simulink model "MANUAL_INTEGRATION_TEST_01"  (Simulink 8.1)
settings: Solver=ode4  StartTime=0.0  StopTime=inf  FixedStep=Ts  MaxStep=1e-3  RelTol=1e-3
model workspace (MAT data in the model file):
  op_snapshot1 : opcond.OperatingPoint (value not decoded)
PostLoadFcn:
  | INTEGRATION_TEST_01_init;
InitFcn:
  | INTEGRATION_TEST_01_init;
values from neighbouring files (symbols this model uses):
  CMD_signals = [1 2 3 4 5 6 7 8 9 10 11 12 ... (1568 elements, 49x32)]    [CMD_signals.mat]
undefined symbols (not defined in the file or in its folder): cable_spec, DiscIntNeverNeededParam, fdesignblkfcn, gcbh, Generator, Left, NG_CHP, NG_CHP_lib, NG_Genset_lib, ph, relay_par, SIM_HIL, Ts, type, V
libraries: simulink x29, rtio_opalrt_common x21, rtlab x7, powerlib_extras x7, simulink_extras x7, cables_lib x6, breaker_lib x4, rtio_generic_modbus x4, powerlib x4, rteventslib x4, Load_lib x3, ssn_lib x2
(part 1 of 4)
settings Model: ARTEMISmethode_block_infos=$$__separator__$$MANUAL_INTEGRATION_TEST_01/ARTEMIS Guide$$__separator__$$  Creator=RE25624  LastModifiedBy=RE25624  BufferReuse=off
settings SolverCC: ZeroCrossAlgorithm=Adaptive
settings DataIOCC: ExternalInput=getinputstruct(op_snapshot1)  InitialState=getstatestruct(op_snapshot1)  LimitDataPoints=off  MaxDataPoints=90060  SignalLoggingSaveFormat=Dataset  SaveOutput=off  SignalLogging=off  DSMLogging=off  SaveTime=off  OutputSaveName=result
settings OptimizationCC: BlockReduction=off  OptimizeBlockIOStorage=off  BufferReuse=off  ExpressionFolding=off  LocalBlockOutputs=off
settings DebuggingCC: MaxConsecutiveZCsMsg=warning  IgnoredZcDiagnostic=none  SolverPrmCheckMsg=none  MultiTaskRateTransMsg=warning  FcnCallInpInsideContextMsg=EnableAllAsWarning  FrameProcessingCompatibilityMsg=error  ModelReferenceExtraNoncontSigs=warning  StrictBusMsg=None
settings ModelReferenceCC: UpdateModelReferenceTargets=IfOutOfDate
settings SFSimCC: SFSimEcho=off
settings GRTTargetCC: CodeReplacementLibrary=C89/C90 (ANSI)

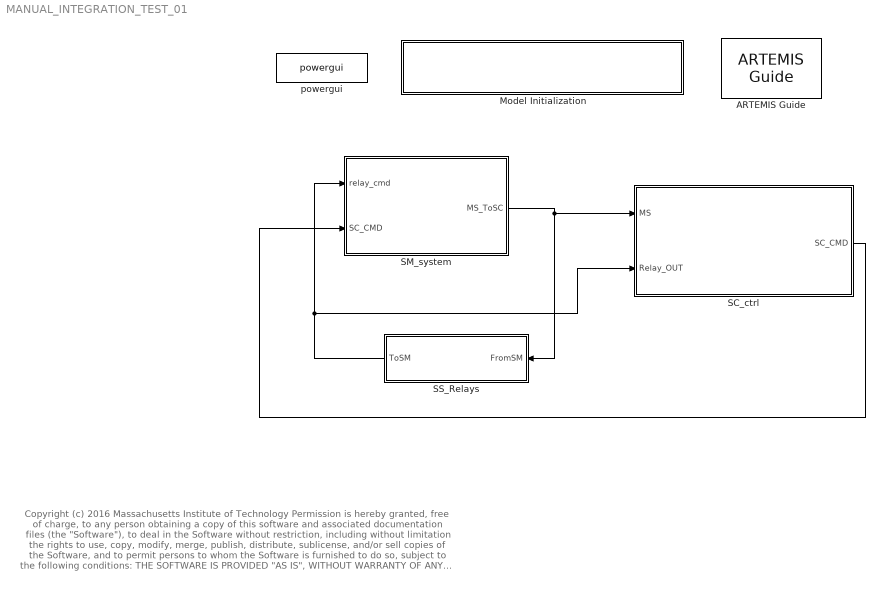
== system MANUAL_INTEGRATION_TEST_01 ==
  note: Copyright (c) 2016 Massachusetts Institute of Technology
      | Permission is hereby granted, free of charge, to any person obtaining a copy of this software and associated documentation files (the "Software"), to deal
      | in the Software without restriction, including without limitation the rights to use, copy, modify, merge, publish, distribute, sublicense, and/or sell copies of the
      | Software, and to permit persons to whom the Software is furnished to do so, subject to the following conditions:
      |
      | THE SOFTWARE IS PROVIDED "AS IS", WITHOUT WARRANTY OF ANY KIND, EXPRESS OR IMPLIED, INCLUDING BUT NOT LIMITED TO THE
      | WARRANTIES OF MERCHANTABILITY, FITNESS FOR A PARTICULAR PURPOSE AND NONINFRINGEMENT. IN NO EVENT SHALL THE AUTHORS
      | OR COPYRIGHT HOLDERS BE LIABLE FOR ANY CLAIM, DAMAGES OR OTHER LIABILITY, WHETHER IN AN ACTION OF CONTRACT, TORT OR
      | OTHERWISE, ARISING FROM, OUT OF OR IN CONNECTION WITH THE SOFTWARE OR THE USE OR OTHER DEALINGS IN THE SOFTWARE.
  ARTEMIS Guide : artemis/ARTEMIS/ARTEMIS Guide  Tag=FTSSmethode_opal_4hx0r99  Description=5.0_z1  lock=on  Ts=Ts  opt=art5  dyna=off  nb_perm=4  RT_fullcomp=off  ssn=on  ssn_itvc=off  ssn_ivic=off  ssn_ext=off  ssn_solver=Art5 with Backward Euler nodal interface  ssn_impulse=off  ssn_quasimpulse=off  ssn_impulse_loop=2  paraExtinctionThy=off  Thy_Impulse=on  dtc=Off  dtc_opt=normal  ao=on  simtype=off  ct_mac=off  lin_mov=off  lsp=[0.001 2]  spike_skip=Disabled  dtc_extra=1  dtc_sws=normal  dtc_pied=0.5  SPSRulesBlock=SPSRules  tre=on  ctmm=off  LF=off  dpl_type=ARTEMiS DPL  rlc_type=off  custom_type=off  para=on  ssn_ImpulseLoopBlockedStateUpdate=2  ssn_mov_iter_number=5  ssn_switch_iter_number=5
  Model Initialization : Subsystem  AncestorBlock=artemis/Tools /Misc/Model Initialization  mask(Model Functions){InitFcnX=INTEGRATION_TEST_01_init;, prel=off, posl=on, inif=on, strf=off}
      mask prompts: InitFcnX "Initialisation"; prel "Preload Function"; posl "PostLoad Function"; inif "InitFcn"; strf "StartFcn"
      mask init:
      | currentBlock = gcb;
      | root = bdroot(currentBlock);
      | 
      | 
      | if ~strcmp(get_param(root,'BlockDiagramType'),'library')
      |     if prel==1
      |         set_param(root, 'PreLoadFcn', InitFcnX);
      |     else
      |         set_param(root, 'PreLoadFcn', '');
      |     end
      |     if inif==1
      |         set_param(root, 'InitFcn', InitFcnX);
      |     else
      |         set_param(root, 'InitFcn', '');
      |     end
      |     if strf==1
      |         set_param(root, 'StartFcn', InitFcnX);
      |     else
      |         set_param(root, 'StartFcn', '');
      |     end
      |     if posl==1
      |         set_param(root, 'PostLoadFcn', InitFcnX);
      |     else
      |         set_param(root, 'PostLoadFcn', '');
      |     end
      | end
      | 
      | pos = get_param(currentBlock, 'Position');
      | width = pos(3) - pos(1); height = pos(4) - pos(2);
      | txt = [ upper(root) '\n' '- InitFcn. . . . . '  get_param(root, 'InitFcn') ];
      settings: CopyFcn=set_param(gcb,'LinkStatus','inactive')
      mask Display: text(5, height*0.5, txt, 'horizontalAlignment', 'left', 'verticalAlignment', 'middle') ;
  SC_ctrl : Subsystem
  SM_system : Subsystem
  SS_Relays : Subsystem
  powergui : powerlib/powergui  Priority=2  SimulationMode=Discrete  SolverType=Tustin  SampleTime=Ts  frequency=60  SPID=off  DisableSnubberDevices=off  DisableRonSwitches=off  DisableVfSwitches=off  SwTol=0  Interpol=off  DisplayEquations=off  frequencyindice=0  Pbase=100e6  ErrMax=1e-4  Iterations=50  UnitsV=kV  UnitsW=MW  FunctionMessages=off  echomessages=off  HookPort=off  EnableUseOfTLC=off  x0status=blocks  RestoreLinks=warning  ResistiveCurrentMeasurement=off  Frange=logspace(0,3,50)  Ylog=off  Xlog=off  ShowGrid=off  save=off  variable=ZData  structure=0  ZoomFFT=on  StartTime=0.0  cycles=2  DisplayStyle=off  fundamental=60  FreqAxis=off  MaxFrequency=1000  frequencyindicesteady=1  RmsSteady=1  display=off  Ts=0  methode=off
  wires:
  SM_system/1(MS_ToSC) -> SC_ctrl/1(MS), SS_Relays/1(FromSM)
  SS_Relays/1(ToSM) -> SM_system/1(relay_cmd), SC_ctrl/2(Relay_OUT)
  SC_ctrl/1(SC_CMD) -> SM_system/2(SC_CMD)

== system MANUAL_INTEGRATION_TEST_01/Model Initialization ==

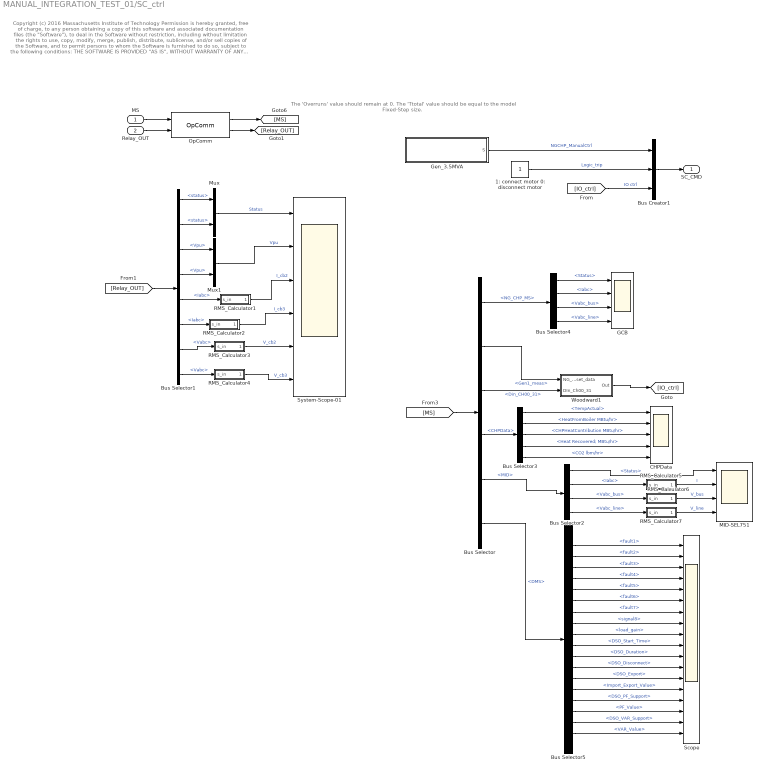
== system MANUAL_INTEGRATION_TEST_01/SC_ctrl ==
  note: The 'Overruns' value should remain at 0.
      | The 'Ttotal' value should be equal to the
      | model Fixed-Step size.
  note: Copyright (c) 2016 Massachusetts Institute of Technology
      | Permission is hereby granted, free of charge, to any person obtaining a copy of this software and associated documentation files (the "Software"), to deal
      | in the Software without restriction, including without limitation the rights to use, copy, modify, merge, publish, distribute, sublicense, and/or sell copies of the
      | Software, and to permit persons to whom the Software is furnished to do so, subject to the following conditions:
      |
      | THE SOFTWARE IS PROVIDED "AS IS", WITHOUT WARRANTY OF ANY KIND, EXPRESS OR IMPLIED, INCLUDING BUT NOT LIMITED TO THE
      | WARRANTIES OF MERCHANTABILITY, FITNESS FOR A PARTICULAR PURPOSE AND NONINFRINGEMENT. IN NO EVENT SHALL THE AUTHORS
      | OR COPYRIGHT HOLDERS BE LIABLE FOR ANY CLAIM, DAMAGES OR OTHER LIABILITY, WHETHER IN AN ACTION OF CONTRACT, TORT OR
      | OTHERWISE, ARISING FROM, OUT OF OR IN CONNECTION WITH THE SOFTWARE OR THE USE OR OTHER DEALINGS IN THE SOFTWARE
  MS : Inport
  Relay_OUT : Inport  Port=2
  1: connect motor 0: disconnect motor : Constant
  Bus Creator1 : BusCreator  Inputs=3
  Bus Selector : BusSelector  OutputSignals=NG_CHP_MS,NG_CHP_MS.Gen1_meas,NG_CHP_MS.Din_CH00_31,NG_CHP_MS.CHPData,MID,DMS
  Bus Selector1 : BusSelector  OutputSignals=CB2.m.status,CB3.m.status,CB2.m.Vpu,CB3.m.Vpu,CB2.m.Iabc,CB3.m.Iabc,CB2.m.Vabc,CB3.m.Vabc
  Bus Selector2 : BusSelector  OutputSignals=Status,Iabc,Vabc_bus,Vabc_line
  Bus Selector3 : BusSelector  OutputSignals=TempActual,HeatFromBoiler MBtu/hr,CHPHeatContribution MBtu/hr,Thermal data.Heat Recovered; MBtu/hr,Thermal data.CO2 lbm/hr
  Bus Selector4 : BusSelector  OutputSignals=NG_CHP_MS.Status,NG_CHP_MS.Iabc,NG_CHP_MS.Vabc_bus,NG_CHP_MS.Vabc_line
  Bus Selector5 : BusSelector  OutputSignals=fault1,fault2,fault3,fault4,fault5,fault6,fault7,signal8,load_gain,DSO_Start_Time,DSO_Duration,DSO_Disconnect,DSO_Export,Import_Export_Value,DSO_PF_Support,PF_Value,DSO_VAR_Support,VAR_Value
  CHPData : Scope  NumInputPorts=5
      settings: ShowLegends=on  TimeRange=10  YMin=20~0~-1~1.37518~932.98  YMax=20.05~5.5~1~1.37533~933.08  SaveName=ScopeData5
  GCB : Scope  NumInputPorts=4
      settings: ShowLegends=on  TimeRange=0.016  YMin=0.95~-800~-12500~-12500  YMax=1.05~800~12500~12500
  Gen_3.5MVA : Subsystem
  MID-SEL751 : Scope  NumInputPorts=4
      settings: ShowLegends=on  TimeRange=0.016  YMin=0.95~-500~-12500~-12500  YMax=1.05~600~12500~12500  SaveName=ScopeData2
  Mux : Mux  Inputs=2
  Mux1 : Mux  Inputs=2
  OpComm : rtlab/OpComm  nbport=2  groupe_acq=1  subsys_rate=0  st=0  Synchronization=on  Interpolation=on  Threshold=1.0  Missed_Data=off  Sim_Time=off  Samples=off  dynSigOut=off  from_console=0  warning_done=off  writeOpCommFile=off  Offset=off
  RMS_Calculator1 : Subsystem
  RMS_Calculator2 : Subsystem
  RMS_Calculator3 : Subsystem
  RMS_Calculator4 : Subsystem
  RMS_Calculator5 : Subsystem
  RMS_Calculator6 : Subsystem
  RMS_Calculator7 : Subsystem
  Scope : Scope  NumInputPorts=18
      settings: YMin=0~0~-1~-1~-1~-1~-1~-1~0.4~0~-5~-5~-5~-5~-5~-5~-5~-5  YMax=1~1~1~1~1~1~1~1~1~4000~5~5~5~5~5~5~5~5  SaveName=ScopeData8  Decimation=100
  System-Scope-01 : Scope  NumInputPorts=6
      settings: ShowLegends=on  TimeRange=1  YMin=0~0~-100~-150~-15000~-15000  YMax=3~1.5~100~150~15000~15000
  Woodward1 : Subsystem
  SC_CMD : Outport
  wires:
  OpComm/1 -> [MS]
  MS/1 -> OpComm/1
  OpComm/2 -> [Relay_OUT]
  Relay_OUT/1 -> OpComm/2
  Woodward1/1(Out) -> [IO_ctrl]
  Bus Selector4/1 -> GCB/1  "<Status>"
  Bus Selector4/2 -> GCB/2  "<Iabc>"
  Bus Selector4/3 -> GCB/3  "<Vabc_bus>"
  Bus Selector4/4 -> GCB/4  "<Vabc_line>"
  Bus Selector/1 -> Bus Selector4/1  "<NG_CHP_MS>"
  Bus Selector/2 -> Woodward1/1(NG_genset_data)  "<Gen1_meas>"
  Bus Selector/3 -> Woodward1/2(DIn_Ch00_31)  "<Din_CH00_31>"
  [MS] -> Bus Selector/1
  Bus Selector/4 -> Bus Selector3/1  "<CHPData>"
  Bus Selector3/1 -> CHPData/1  "<TempActual>"
  Bus Selector3/5 -> CHPData/5  "<CO2 lbm/hr>"
  Bus Selector3/2 -> CHPData/2  "<HeatFromBoiler MBtu/hr>"
  Bus Selector3/3 -> CHPData/3  "<CHPHeatContribution MBtu/hr>"
  Bus Selector3/4 -> CHPData/4  "<Heat Recovered; MBtu/hr>"
  [Relay_OUT] -> Bus Selector1/1
  Bus Selector1/1 -> Mux/1  "<status>"
  Bus Selector1/2 -> Mux/2  "<status>"
  Bus Selector1/3 -> Mux1/1  "<Vpu>"
  Bus Selector1/4 -> Mux1/2  "<Vpu>"
  Bus Creator1/1 -> SC_CMD/1
  1: connect motor 0: disconnect motor/1 -> Bus Creator1/2  "Logic_trip"
  [IO_ctrl] -> Bus Creator1/3  "IO ctrl"
  Gen_3.5MVA/1(S) -> Bus Creator1/1  "NGCHP_ManualCtrl"
  Mux/1 -> System-Scope-01/1  "Status"
  Mux1/1 -> System-Scope-01/2  "Vpu"
  Bus Selector1/5 -> RMS_Calculator1/1(s_in)  "<Iabc>"
  Bus Selector1/6 -> RMS_Calculator2/1(s_in)  "<Iabc>"
  RMS_Calculator1/1(s_out) -> System-Scope-01/3  "I_cb2"
  RMS_Calculator2/1(s_out) -> System-Scope-01/4  "I_cb3"
  Bus Selector1/7 -> RMS_Calculator3/1(s_in)  "<Vabc>"
  Bus Selector1/8 -> RMS_Calculator4/1(s_in)  "<Vabc>"
  RMS_Calculator3/1(s_out) -> System-Scope-01/5  "V_cb2"
  RMS_Calculator4/1(s_out) -> System-Scope-01/6  "V_cb3"
  Bus Selector2/1 -> MID-SEL751/1  "<Status>"
  Bus Selector2/2 -> RMS_Calculator5/1(s_in)  "<Iabc>"
  Bus Selector2/3 -> RMS_Calculator6/1(s_in)  "<Vabc_bus>"
  Bus Selector2/4 -> RMS_Calculator7/1(s_in)  "<Vabc_line>"
  Bus Selector/5 -> Bus Selector2/1  "<MID>"
  RMS_Calculator5/1(s_out) -> MID-SEL751/2  "I"
  RMS_Calculator6/1(s_out) -> MID-SEL751/3  "V_bus"
  RMS_Calculator7/1(s_out) -> MID-SEL751/4  "V_line"
  Bus Selector/6 -> Bus Selector5/1  "<DMS>"
  Bus Selector5/1 -> Scope/1  "<fault1>"
  Bus Selector5/2 -> Scope/2  "<fault2>"
  Bus Selector5/3 -> Scope/3  "<fault3>"
  Bus Selector5/4 -> Scope/4  "<fault4>"
  Bus Selector5/5 -> Scope/5  "<fault5>"
  Bus Selector5/6 -> Scope/6  "<fault6>"
  Bus Selector5/7 -> Scope/7  "<fault7>"
  Bus Selector5/8 -> Scope/8  "<signal8>"
  Bus Selector5/9 -> Scope/9  "<load_gain>"
  Bus Selector5/10 -> Scope/10  "<DSO_Start_Time>"
  Bus Selector5/11 -> Scope/11  "<DSO_Duration>"
  Bus Selector5/12 -> Scope/12  "<DSO_Disconnect>"
  Bus Selector5/13 -> Scope/13  "<DSO_Export>"
  Bus Selector5/14 -> Scope/14  "<Import_Export_Value>"
  Bus Selector5/15 -> Scope/15  "<DSO_PF_Support>"
  Bus Selector5/16 -> Scope/16  "<PF_Value>"
  Bus Selector5/17 -> Scope/17  "<DSO_VAR_Support>"
  Bus Selector5/18 -> Scope/18  "<VAR_Value>"

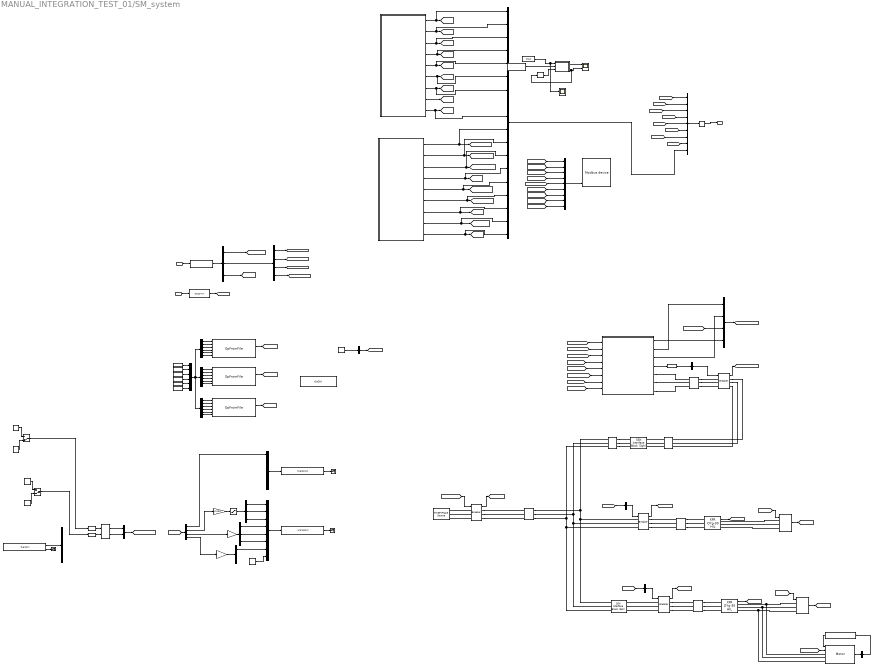
== system MANUAL_INTEGRATION_TEST_01/SM_system ==
  note: Copyright (c) 2016 Massachusetts Institute of Technology
      | Permission is hereby granted, free of charge, to any person obtaining a copy of this software and associated documentation files (the "Software"), to deal
      | in the Software without restriction, including without limitation the rights to use, copy, modify, merge, publish, distribute, sublicense, and/or sell copies of the
      | Software, and to permit persons to whom the Software is furnished to do so, subject to the following conditions:
      |
      | THE SOFTWARE IS PROVIDED "AS IS", WITHOUT WARRANTY OF ANY KIND, EXPRESS OR IMPLIED, INCLUDING BUT NOT LIMITED TO THE
      | WARRANTIES OF MERCHANTABILITY, FITNESS FOR A PARTICULAR PURPOSE AND NONINFRINGEMENT. IN NO EVENT SHALL THE AUTHORS
      | OR COPYRIGHT HOLDERS BE LIABLE FOR ANY CLAIM, DAMAGES OR OTHER LIABILITY, WHETHER IN AN ACTION OF CONTRACT, TORT OR
      | OTHERWISE, ARISING FROM, OUT OF OR IN CONNECTION WITH THE SOFTWARE OR THE USE OR OTHER DEALINGS IN THE SOFTWARE
  note: Stop_index = length of data - 1 to data chopping
  note: This connector also services Genset #2 and  is
      | shared with Genset #1.  Use RJ45 connectors to
      |  intercept Genset #2 I/O (not used in this Device
      | Integration Test) and use for SEL-751
  note: Remove existing connections to Slot 3 I/O, if any
      | ans replace with connections shown below, or use
      | corresponding RJ45 connectors.  (Existing I/O, if any not
      |  used for this Device Integration Test)
  note: This Modbus slave device makes the DMS
      | commands available to the MGC via a Modbus
      | slave
  note: This embedded script updates model
      | parameters and DMS commands based
      | on a predetermined schedule.
  relay_cmd : Inport
  SC_CMD : Inport  Port=2
  200 HP chiller compressor : Load_lib/200 HP chiller compressor
  AnalogOut2 to SEL-751 : rtio_opalrt_common/AnalogOut  CtrlName='OpCtrl'  portNb=4  FcnNos=Slot 2 Module A Subsection 2  size=16  maxcount=8  count=8  numchan=8  israngeinput=off  voltagerange=[ -5 ... 5 ]  slot=1  side=0  mismatch=0  slotside=Slot_2_Module_A
      settings: AttributesFormatString=%<CtrlName>
  Bus Creator : BusCreator  Inputs=9
  Bus Creator1 : BusCreator
  Bus Creator2 : BusCreator  Inputs=1
  Bus Creator3 : BusCreator  Inputs=1
  Bus Creator4 : BusCreator  Inputs=2
  Bus Creator5 : BusCreator  Inputs=18
  Bus Selector1 : BusSelector  OutputSignals=CB2
  Bus Selector2 : BusSelector  OutputSignals=CB3
  Bus Selector3 : BusSelector  OutputSignals=NGCHP_ManualCtrl,IO ctrl,Logic_trip
  Bus Selector4 : BusSelector  OutputSignals=Status,Iabc,Vabc_line,Vabc_bus
  Bus Selector5 : BusSelector  OutputSignals=Woodward,manual_controls,DOUT GR3,DOUT GR3.16 DOUT GR3.CHP_SIM_Cmds
  Bus Selector6 : BusSelector  OutputSignals=RPM
  CB closed : Constant
  CB1-GCB1 : breaker_lib/Breaker  Ts=Ts  mech_delay=cb_mech_delay
  CB2 : breaker_lib/Breaker  Ts=Ts  mech_delay=cb_mech_delay
  CB3 : breaker_lib/Breaker  Ts=Ts  mech_delay=cb_mech_delay
  CT Ratio : Gain  Gain=5/1250
  Cal : Constant  Value=0
  Constant : Constant
  Constant1 : Constant  Value=0
  Constant2 : Constant
  Constant3 : Constant  Value=0
  DMS Modbus  device : rtio_generic_modbus/Modbus device  conf_name=DMS_slave_cfg.opal  conf_name_mask=DMS_slave_cfg.xls  sample_time=0
  DMSCommandsToMGC : Subsystem  mask{DSO_Start_Time=3600, DSO_Duration=0, DSO_Disconnect=1, DSO_Export=0, Import_Export_Value=0, DSO_PF_Support=0, PF_Value=0, DSO_VAR_Support=0, VAR_Value=0}
      mask prompts: DSO_Start_Time "DSO Start Time"; DSO_Duration "DSO Duration"; DSO_Disconnect "DSO Disconnect"; DSO_Export "DSO Export (1) or Import (0)"; Import_Export_Value "Import/Export Value, kW"; DSO_PF_Support "DSO PF Support (1) or Not (0)"; PF_Value "PF Value, pu, "+"(lagging) "-" (leading)"; DSO_VAR_Support "DSO VAR Support (1) or Not (0)"; VAR_Value "Import/Export Value, kVAr"
  Data Type Conversion : DataTypeConversion
  Data Type Conversion1 : DataTypeConversion
  Demux : Demux  Outputs=3
  Demux1 : Demux  Outputs=6
  Demux2 : Demux  Outputs=6
  Demux3 : Demux  Outputs=6
  Demux4 : Demux  Outputs=3
  Demux5 : Demux  Outputs=3
  Demux6 : Demux  Outputs=8
  Digital Clock : DigitalClock  SampleTime=Ts
  DigitalIn from SEL-751 : rtio_opalrt_common/DigitalIn  CtrlName='OpCtrl'  portNb=6  FcnNos=Slot 3 Module A Subsection 2  size=1  maxcount=8  count=8  sampleTime=Ts  numchan=8
      settings: AttributesFormatString=%<CtrlName>
  DigitalOut to SEL-751 : rtio_opalrt_common/DigitalOut  CtrlName='OpCtrl'  portNb=6  FcnNos=Slot 3 Module B Subsection 2  size=1  maxcount=8  count=8  numchan=8
      settings: AttributesFormatString=%<CtrlName>
  Dynamic_Load_1 : Load_lib/Dynamic_Load  V=4160  Ts=Ts
  Dynamic_Load_2 : Load_lib/Dynamic_Load  V=480  Ts=Ts
  Fcn : Fcn  Expr=u(1)==1
  GRID : powerlib/Electrical Sources/Three-Phase Source  Voltage=13800  PhaseAngle=0  Frequency=60  InternalConnection=Yg  SpecifyImpedance=on  Resistance=0.8929  Inductance=16.58e-3  ShortCircuitLevel=375e6  BaseVoltage=13800  XRratio=4.6  BusType=swing  Pref=0  Qref=0  Qmin=-inf  Qmax=inf
  "Interpolation " : Constant
  MID : breaker_lib/Breaker  Ts=Ts  mech_delay=cb_mech_delay
  Manual Switch : ManualSwitch  CurrentSetting=0
  Manual Switch1 : ManualSwitch  CurrentSetting=0
  Memory : Memory
  Memory1 : Memory  X0=1
  Motor : Motor_InductionMachine_lib/Motor
  Mux : Mux  Inputs=6
  Mux1 : Mux  Inputs=8
  Mux2 : Mux  Inputs=9
  Mux4 : Mux  Inputs=8
  NG_CHP1 : Subsystem  AncestorBlock=NG_CHP_lib/NG_CHP
  OpComm : rtlab/OpComm  nbport=1  groupe_acq=1  subsys_rate=0  st=0  Synchronization=on  Interpolation=on  Threshold=1.0  Missed_Data=off  Sim_Time=off  Samples=off  dynSigOut=off  from_console=0  warning_done=off  writeOpCommFile=off  Offset=off
  OpComm2 : rtlab/OpComm  nbport=1  groupe_acq=1  subsys_rate=0  st=0  Synchronization=on  Interpolation=on  Threshold=1.0  Missed_Data=off  Sim_Time=off  Samples=off  dynSigOut=off  from_console=1  warning_done=off  writeOpCommFile=off  Offset=off
  OpCtrl : rtio_opalrt_common/OpCtrl  CtrlName='OpCtrl'  boardid=0  BitstreamFilename=VC707_2-EX-0001-2_2_6_61-32AIO16DIO16DIOSel-01-01.bin  numconfig=-1  mode=Master  externalClock=off  decimRtsi=0  calibIO=off  SampleTime=0  loadinport=-1  BoardType=VC707  SecondaryPresent=off  sync_type=Audio
  OpFromFile : rtlab/DataLogging/OpFromFile  filename_mode=Static (same filename all the time)  reload_mode=Next time model is paused (Real-Time)  init_file_id=0  filename=HeatLoad.mat  rtpath='./'  nrtpath='.\'  sample_time=Ts
  OpFromFile1 : rtlab/DataLogging/OpFromFile  filename_mode=Static (same filename all the time)  reload_mode=Next time model is paused (Real-Time)  init_file_id=0  filename=one_min_data.mat  rtpath='./'  nrtpath='.\'  sample_time=0
  OpFromFile2 : rtlab/DataLogging/OpFromFile  filename_mode=Static (same filename all the time)  reload_mode=Next time model is paused (Real-Time)  init_file_id=0  filename=one_min_data.mat  rtpath='./'  nrtpath='.\'  sample_time=0
  PI-Section : cables_lib/PI-Section  cable_spec=[cable_spec(13, :)]  line_length=5500  parallel_sets=1
  PI-Section1 : cables_lib/PI-Section  cable_spec=[cable_spec(11, :)]  line_length=10  parallel_sets=1
  PI-Section2 : cables_lib/PI-Section  cable_spec=[cable_spec(11, :)]  line_length=2000  parallel_sets=1
  PI-Section3 : cables_lib/PI-Section  cable_spec=[cable_spec(13, :)]  line_length=1500  parallel_sets=1
  PI-Section4 : cables_lib/PI-Section  cable_spec=[cable_spec(13, :)]  line_length=2000  parallel_sets=1
  PI-Section5 : cables_lib/PI-Section  cable_spec=[cable_spec(11, :)]  line_length=10  parallel_sets=1
  PT Ratio1 : Gain  Gain=1/1800
  PT Ratio2 : Gain  Gain=1/1800
  "Repetative " : Constant
  S-R Flip-Flop : simulink_extras/Flip Flops/S-R Flip-Flop  initial_condition=1
  SSN Interface Block (3ph) : ssn_lib/SSN Interface Block (3ph)  nb_phase=3  nb_port=2  p1_type=V-type(Left)  p2_type=V-type (Right)  p3_type=V-type(Left)  p4_type=V-type(Left)  p5_type=V-type(Left)  p6_type=V-type(Left)  p7_type=V-type(Left)  p8_type=V-type(Left)  p9_type=V-type(Left)  p10_type=V-type(Left)  p11_type=V-type(Left)  p12_type=V-type(Left)  p13_type=V-type(Left)  p14_type=V-type(Left)  p15_type=V-type(Left)  p16_type=V-type(Left)  I_port_shunt_resistance=1e9
  SSN Interface Block (3ph)1 : ssn_lib/SSN Interface Block (3ph)  nb_phase=3  nb_port=2  p1_type=V-type(Left)  p2_type=V-type (Right)  p3_type=V-type(Left)  p4_type=V-type(Left)  p5_type=V-type(Left)  p6_type=V-type(Left)  p7_type=V-type(Left)  p8_type=V-type(Left)  p9_type=V-type(Left)  p10_type=V-type(Left)  p11_type=V-type(Left)  p12_type=V-type(Left)  p13_type=V-type(Left)  p14_type=V-type(Left)  p15_type=V-type(Left)  p16_type=V-type(Left)  I_port_shunt_resistance=1e9
  Scheduler : MATLAB Function  TreatAsAtomicUnit=on
  Scope1 : Scope
      settings: YMin=1.04083e-17  YMax=0.2  SaveName=ScopeData6
  Scope4 : Scope  NumInputPorts=3
      settings: YMin=-5~-5~-5  YMax=5~5~5  SaveName=ScopeData7
  "Start_Index " : Constant
  "State " : Constant
  "Stop_Index " : Constant  Value=1800-1
  Terminator : Terminator
  Terminator1 : Terminator
  Terminator2 : Terminator
  Test Sequence Inputs : Constant  Value=CMD_signals
  TestSequenceCommands : Subsystem  mask{fault1=0, fault2=0, fault3=0, fault4=0, fault5=0, fault6=0, fault7=0, fault8=0, load_gain=0.5}
      mask prompts: load_gain "Loads"
  Thermal Protection for Transconductance Amp : Saturate  UpperLimit=5  LowerLimit=-5
  "Time_Scale_Factor " : Constant
  XFR DYg-30 HIL1 : transformer_lib/XFR DYg-30 HIL  Rating=3750  Vp=13800  Vs=4160  Z=4.75  XR=11.4
  XFR DYg-30 HIL2 : transformer_lib/XFR DYg-30 HIL  Rating=2500  Vp=13800  Vs=480  Z=5.75  XR=6.6
  MS_ToSC : Outport
  wires:
  MID/1 -> [MID]
  Bus Creator/1 -> Memory/1
  OpComm/1 -> [relay_cmd]
  relay_cmd/1 -> OpComm/1
  CB1-GCB1/1 -> [NG_CHP_GCB]
  SC_CMD/1 -> OpComm2/1
  Bus Selector5/1 -> [woodward]  "<Woodward>"
  Bus Selector5/3 -> [Dout_GR3]  "<DOUT GR3>"
  Bus Selector5/2 -> [brkcont]  "<manual_controls>"
  [NG_CHP_GCB] -> Bus Creator1/3  "NG_CHP_MS"
  NG_CHP1/3(Generator Data) -> Bus Creator1/2  "Gen1_meas"
  NG_CHP1/2(Out2) -> Bus Creator1/1  "Din_CH00_31"
  XFR DYg-30 HIL1/1 -> [XFR_01]
  "Stop_Index "/1 -> Mux/4
  Demux1/2 -> OpFromFile1/2
  Demux1/5 -> OpFromFile1/5
  OpFromFile1/2 -> [PQLOAD_2]
  "Interpolation "/1 -> Mux/6
  Demux1/4 -> OpFromFile1/4
  Demux1/1 -> OpFromFile1/1
  Demux1/6 -> OpFromFile1/6
  Demux1/3 -> OpFromFile1/3
  "Start_Index "/1 -> Mux/3
  "Time_Scale_Factor "/1 -> Mux/5
  "Repetative "/1 -> Mux/2
  "State "/1 -> Mux/1
  [Dout_GR3] -> NG_CHP1/2(Digital Outputs)
  [brkcont] -> NG_CHP1/3(Console Breakers)
  [woodward] -> NG_CHP1/4(Woodward Enable)
  [NGCHP_MNCTLR] -> NG_CHP1/5(Manual Control (opt))
  [NG_CHP_GCB] -> NG_CHP1/6(GCB)
  [MID] -> NG_CHP1/7(MCB)
  NG_CHP1/1(Out1) -> Bus Creator1/4  "CHPData"
  NG_CHP1/4(GCB Control) -> Fcn/1
  Bus Selector5/4 -> [CHP_SIM_cmds]  "<CHP_SIM_Cmds>"
  OpFromFile/2 -> [heat_load]  "Heat Load MBtu/hr"
  [heat_load] -> NG_CHP1/1(In1)
  [CHP_SIM_cmds] -> NG_CHP1/8(In2)
  Demux2/2 -> OpFromFile/2
  Demux2/5 -> OpFromFile/5
  Demux2/4 -> OpFromFile/4
  Demux2/1 -> OpFromFile/1
  Demux2/6 -> OpFromFile/6
  Demux2/3 -> OpFromFile/3
  Dynamic_Load_1/1 -> [LOAD_1]
  XFR DYg-30 HIL2/1 -> [XFR_02]
  Dynamic_Load_2/1 -> [LOAD_2]
  Bus Creator2/1 -> [cb_c]
  CB closed/1 -> Bus Creator2/1  "Logic_trip"
  CB2/1 -> [CB2]
  CB3/1 -> [CB3]
  [XFR_02] -> Bus Creator/7  "XFR_02"
  [LOAD_2] -> Bus Creator/5  "LOAD_2"
  [XFR_01] -> Bus Creator/6  "XFR_01"
  [MID] -> Bus Creator/1  "MID"
  [CB3] -> Bus Creator/3  "CB3"
  [CB2] -> Bus Creator/2  "CB2"
  [LOAD_1] -> Bus Creator/4  "LOAD_1"
  Bus Creator1/1 -> [NG_CHP_MS]
  [NG_CHP_MS] -> Bus Creator/8  "NG_CHP_MS"
  Demux3/2 -> OpFromFile2/2
  Demux3/5 -> OpFromFile2/5
  OpFromFile2/2 -> [PQLOAD_1]
  Demux3/4 -> OpFromFile2/4
  Demux3/1 -> OpFromFile2/1
  Demux3/6 -> OpFromFile2/6
  Demux3/3 -> OpFromFile2/3
  Mux/1 -> Demux3/1, Demux2/1, Demux1/1
  [PQLOAD_1] -> Dynamic_Load_1/1
  [PQLOAD_2] -> Dynamic_Load_2/1
  [relay_cmd] -> Bus Selector1/1
  Bus Selector1/1 -> CB2/1  "<CB2>"
  [relay_cmd] -> Bus Selector2/1
  Bus Selector2/1 -> CB3/1  "<CB3>"
  Fcn/1 -> Bus Creator3/1  "Logic_trip"
  Bus Creator3/1 -> CB1-GCB1/1  "Logic_trip"
  [SEL751_1_from] -> MID/1
  [motor_cmd] -> Motor/2
  Motor/1 -> Bus Selector6/1
  Bus Selector6/1 -> 200 HP chiller compressor/1  "<RPM>"
  200 HP chiller compressor/1 -> Motor/1
  OpComm2/1 -> Bus Selector3/1
  Bus Selector3/1 -> [NGCHP_MNCTLR]  "<NGCHP_ManualCtrl>"
  Bus Selector3/2 -> Bus Selector5/1  "<IO ctrl>"
  Bus Selector3/3 -> [motor_cmd]  "<Logic_trip>"
  Bus Selector4/2 -> CT Ratio/1  "<Iabc>"
  Demux4/1 -> Mux1/4  "Va"
  Demux4/2 -> Mux1/5  "Vb"
  Demux4/3 -> Mux1/6  "Vc"
  Bus Selector4/4 -> PT Ratio2/1  "<Vabc_bus>"
  Demux5/1 -> Mux1/7  "Vs"
  Bus Selector4/3 -> PT Ratio1/1  "<Vabc_line>"
  Cal/1 -> Mux1/8
  AnalogOut2 to SEL-751/1 -> Terminator/1
  DigitalIn from SEL-751/1 -> Demux6/1
  Manual Switch/1 -> Data Type Conversion/1  "OUT103 Brkr trip"
  Manual Switch1/1 -> Data Type Conversion1/1  "OUT102 Brkr reset"
  Data Type Conversion/1 -> S-R Flip-Flop/1
  Data Type Conversion1/1 -> S-R Flip-Flop/2
  S-R Flip-Flop/1 -> Bus Creator4/1  "Logic_trip"
  S-R Flip-Flop/2 -> Bus Creator4/2  "Logic_reset"
  Bus Selector4/1 -> Mux4/1  "<Status>"
  Mux4/1 -> DigitalOut to SEL-751/1
  DigitalOut to SEL-751/1 -> Terminator1/1
  DigitalIn from SEL-751/2 -> Terminator2/1
  Mux1/1 -> AnalogOut2 to SEL-751/1
  Demux/1 -> Mux1/1  "Ia"
  Demux/3 -> Mux1/3  "Ic"
  Demux/2 -> Mux1/2  "Ib"
  Bus Creator4/1 -> [SEL751_1_from]
  [MID] -> Bus Selector4/1
  Memory/1 -> MS_ToSC/1
  Constant1/1 -> Manual Switch/2
  Constant/1 -> Manual Switch/1
  Constant3/1 -> Manual Switch1/2
  Constant2/1 -> Manual Switch1/1
  Mux2/1 -> DMS Modbus  device/4
  Scheduler/1(y) -> Scope4/1
  Scheduler/2(n1) -> Memory1/1, Scope4/3
  Memory1/1 -> Scheduler/3(n)
  Test Sequence Inputs/1 -> Scheduler/2(CMD_signals)
  Digital Clock/1 -> Scheduler/1(u), Scope1/1
  DMSCommandsToMGC/3(DSO_Disconnect) -> Bus Creator5/12, [DSO_Disconnect]
  DMSCommandsToMGC/4(DSO_Export) -> Bus Creator5/13, [DSO_Export]
  DMSCommandsToMGC/7(PF_Value) -> [PF_Value], Bus Creator5/16
  DMSCommandsToMGC/1(DSO_Start_Time) -> [DSO_Start_Time], Bus Creator5/10
  DMSCommandsToMGC/5(Import_Export_Value) -> Bus Creator5/14, [Import_Export_Value]
  [DSO_Start_Time] -> Mux2/1
  [DSO_Duration] -> Mux2/2
  [DSO_Disconnect] -> Mux2/3
  [DSO_Export] -> Mux2/4
  [Import_Export_Value] -> Mux2/5
  [DSO_PF_Support] -> Mux2/6
  [PF_Value] -> Mux2/7
  [DSO_VAR_Support] -> Mux2/8
  [VAR_Value] -> Mux2/9
  TestSequenceCommands/1(Fault1) -> Bus Creator5/1, [fault1]  "fault1"
  TestSequenceCommands/2(Fault2) -> Bus Creator5/2, [fault2]  "fault2"
  TestSequenceCommands/3(Fault3) -> Bus Creator5/3, [fault3]  "fault3"
  TestSequenceCommands/4(Fault4) -> Bus Creator5/4, [fault4]  "fault4"
  TestSequenceCommands/6(Fault6) -> Bus Creator5/6, [fault6]  "fault6"
  TestSequenceCommands/7(Fault7) -> Bus Creator5/7, [fault7]  "fault7"
  TestSequenceCommands/9(loads) -> Bus Creator5/9, [load_gain]  "load_gain"
  TestSequenceCommands/5(Fault5) -> Bus Creator5/5, [fault5]  "fault5"
  DMSCommandsToMGC/2(DSO_Duration) -> Bus Creator5/11, [DSO_Duration]
  DMSCommandsToMGC/6(DSO_PF_Support) -> Bus Creator5/15, [DSO_PF_Support]
  DMSCommandsToMGC/8(DSO_VAR_Support) -> Bus Creator5/17, [DSO_VAR_Support]
  DMSCommandsToMGC/9(VAR_Value) -> Bus Creator5/18, [VAR_Value]
  Bus Creator5/1 -> Bus Creator/9  "DMS"
  TestSequenceCommands/8("Fault8 ") -> [fault8]  "fault8"
  CT Ratio/1 -> Thermal Protection for Transconductance Amp/1
  PT Ratio1/1 -> Demux4/1
  PT Ratio2/1 -> Demux5/1
  Thermal Protection for Transconductance Amp/1 -> Demux/1
  connections:
  Dynamic_Load_1/LConn1 -- XFR DYg-30 HIL1/RConn1
  Dynamic_Load_1/LConn2 -- XFR DYg-30 HIL1/RConn2
  Dynamic_Load_1/LConn3 -- XFR DYg-30 HIL1/RConn3
  CB2/RConn2 -- PI-Section3/LConn2
  CB2/RConn1 -- PI-Section3/LConn1
  CB2/RConn3 -- PI-Section3/LConn3
  CB3/RConn2 -- PI-Section4/LConn2
  CB3/RConn1 -- PI-Section4/LConn1
  CB3/RConn3 -- PI-Section4/LConn3
  CB3/LConn2 -- SSN Interface Block (3ph)/RConn2
  CB3/LConn1 -- SSN Interface Block (3ph)/RConn1
  CB3/LConn3 -- SSN Interface Block (3ph)/RConn3
  PI-Section5/LConn3 -- PI-Section/RConn3 -- SSN Interface Block (3ph)/LConn3 -- CB2/LConn3
  PI-Section5/LConn2 -- PI-Section/RConn2 -- SSN Interface Block (3ph)/LConn2 -- CB2/LConn2
  PI-Section5/LConn1 -- PI-Section/RConn1 -- SSN Interface Block (3ph)/LConn1 -- CB2/LConn1
  Dynamic_Load_2/LConn1 -- Motor/LConn1 -- XFR DYg-30 HIL2/RConn1
  Dynamic_Load_2/LConn3 -- Motor/LConn3 -- XFR DYg-30 HIL2/RConn3
  Dynamic_Load_2/LConn2 -- Motor/LConn2 -- XFR DYg-30 HIL2/RConn2
  PI-Section4/RConn1 -- XFR DYg-30 HIL2/LConn1
  PI-Section4/RConn2 -- XFR DYg-30 HIL2/LConn2
  PI-Section4/RConn3 -- XFR DYg-30 HIL2/LConn3
  PI-Section3/RConn2 -- XFR DYg-30 HIL1/LConn2
  PI-Section3/RConn3 -- XFR DYg-30 HIL1/LConn3
  PI-Section3/RConn1 -- XFR DYg-30 HIL1/LConn1
  PI-Section2/RConn3 -- CB1-GCB1/LConn3
  PI-Section2/RConn2 -- CB1-GCB1/LConn2
  PI-Section2/RConn1 -- CB1-GCB1/LConn1
  NG_CHP1/RConn2 -- PI-Section2/LConn2
  NG_CHP1/RConn3 -- PI-Section2/LConn3
  NG_CHP1/RConn1 -- PI-Section2/LConn1
  PI-Section1/LConn1 -- SSN Interface Block (3ph)1/RConn1
  PI-Section1/LConn2 -- SSN Interface Block (3ph)1/RConn2
  PI-Section1/LConn3 -- SSN Interface Block (3ph)1/RConn3
  PI-Section5/RConn2 -- SSN Interface Block (3ph)1/LConn2
  PI-Section5/RConn1 -- SSN Interface Block (3ph)1/LConn1
  PI-Section5/RConn3 -- SSN Interface Block (3ph)1/LConn3
  CB1-GCB1/RConn3 -- PI-Section1/RConn3
  CB1-GCB1/RConn1 -- PI-Section1/RConn1
  CB1-GCB1/RConn2 -- PI-Section1/RConn2
  MID/RConn3 -- PI-Section/LConn3
  MID/RConn2 -- PI-Section/LConn2
  MID/RConn1 -- PI-Section/LConn1
  MID/LConn3 -- GRID/RConn3
  MID/LConn1 -- GRID/RConn1
  MID/LConn2 -- GRID/RConn2

== system MANUAL_INTEGRATION_TEST_01/SS_Relays ==
  note: Copyright (c) 2016 Massachusetts Institute of Technology
      | Permission is hereby granted, free of charge, to any person obtaining a copy of this software and associated documentation files (the "Software"), to deal
      | in the Software without restriction, including without limitation the rights to use, copy, modify, merge, publish, distribute, sublicense, and/or sell copies of the
      | Software, and to permit persons to whom the Software is furnished to do so, subject to the following conditions:
      |
      | THE SOFTWARE IS PROVIDED "AS IS", WITHOUT WARRANTY OF ANY KIND, EXPRESS OR IMPLIED, INCLUDING BUT NOT LIMITED TO THE
      | WARRANTIES OF MERCHANTABILITY, FITNESS FOR A PARTICULAR PURPOSE AND NONINFRINGEMENT. IN NO EVENT SHALL THE AUTHORS
      | OR COPYRIGHT HOLDERS BE LIABLE FOR ANY CLAIM, DAMAGES OR OTHER LIABILITY, WHETHER IN AN ACTION OF CONTRACT, TORT OR
      | OTHERWISE, ARISING FROM, OUT OF OR IN CONNECTION WITH THE SOFTWARE OR THE USE OR OTHER DEALINGS IN THE SOFTWARE
  FromSM : Inport
  Bus Creator : BusCreator  Inputs=2
  Bus Selector : BusSelector  OutputSignals=CB2,CB3
  Generic_Relay_v2_1 : relay_modbus_lib/Generic_Relay_v2_1  Ts=Ts  relay_settings=[relay_par(1,:)]
  Generic_Relay_v2_2 : relay_modbus_lib/Generic_Relay_v2_1  Ts=Ts  relay_settings=[relay_par(2,:)]
  Memory : Memory
  Modbus device : rtio_generic_modbus/Modbus device  conf_name=F1_relay_cfg1.opal  conf_name_mask=F1_relay_cfg1.xls  sample_time=Ts
  Modbus device1 : rtio_generic_modbus/Modbus device  conf_name=F1_relay_cfg2.opal  conf_name_mask=F1_relay_cfg2.xls  sample_time=Ts
  OpComm : rtlab/OpComm  nbport=1  groupe_acq=1  subsys_rate=0  st=0  Synchronization=on  Interpolation=on  Threshold=1.0  Missed_Data=off  Sim_Time=off  Samples=off  dynSigOut=off  from_console=0  warning_done=off  writeOpCommFile=off  Offset=off
  ToSM : Outport
  wires:
  OpComm/1 -> Bus Selector/1
  FromSM/1 -> OpComm/1
  Generic_Relay_v2_1/1 -> Bus Creator/1  "CB2"
  Generic_Relay_v2_2/1 -> Bus Creator/2  "CB3"
  Bus Creator/1 -> Memory/1
  Modbus device/1 -> Generic_Relay_v2_1/2
  Generic_Relay_v2_1/2 -> Modbus device/1
  Modbus device1/1 -> Generic_Relay_v2_2/2
  Generic_Relay_v2_2/2 -> Modbus device1/1
  Bus Selector/2 -> Generic_Relay_v2_2/1  "<CB3>"
  Bus Selector/1 -> Generic_Relay_v2_1/1  "<CB2>"
  Memory/1 -> ToSM/1

== system MANUAL_INTEGRATION_TEST_01/SC_ctrl/Gen_3.5MVA ==
  1 - PQ 2 - PV 3 - VF : Constant  Value=3
  2.5 - 130 s : DiscretePulseGenerator  Period=150/Ts  PulseWidth=127.5/Ts  PhaseDelay=2.5/Ts  SampleTime=Ts
  Bus Creator : BusCreator  Inputs=6
  DONOTCHANGE : Constant
  Enable = 1 Disable = 0 : Constant  Value=0
  F : simulink/Math Operations/Slider Gain  low=0.97  gain=1  high=1.03
  Fcmd pu 1.005 - 1.03 : Constant  Value=1.005
  P : simulink/Math Operations/Slider Gain  low=0  gain=0.8  high=1.1
  Pfactor : Gain  Gain=.9
  Q : simulink/Math Operations/Slider Gain  low=0.01  gain=0.2  high=0.4
  Qfactor : Gain  Gain=.43
  S Profile : simulink/Sources/Repeating Sequence Stair  OutValues=[.1 .1 .1 .1 .1 .1 .5 .5 .5 .5 .5 .5 .5 .5 .5 .5 .5 .5 1 1 1 1 1 ]  tsamp=[5 Ts]  OutMin=[]  OutMax=[]  OutDataTypeStr=Inherit: Inherit via back propagation  OutDataType=fixdt(0,8)  ConRadixGroup=Best Precision: Vector-wise  OutScaling=2^-12
  V : simulink/Math Operations/Slider Gain  low=0.9  gain=1  high=1.1
  VF - to end : simulink/Sources/Repeating Sequence Stair  OutValues=[3 3 3 3 3 3 3 3 3 3 3 3 3 3 3 3 3 3 3 3 3 3 3 3 3 3 3 3 3 3 3 ]  tsamp=[5 Ts]  OutMin=[]  OutMax=[]  OutDataTypeStr=Inherit: Inherit via back propagation  OutDataType=fixdt(0,8)  ConRadixGroup=Best Precision: Vector-wise  OutScaling=2^-12
  Vcmd pu 1.005 - 1.01 : Constant  Value=1.005
  S : Outport
  wires:
  Pfactor/1 -> Bus Creator/1  "P"
  Fcmd pu 1.005 - 1.03/1 -> Bus Creator/4  "F"
  2.5 - 130 s/1 -> Bus Creator/6  "Enable"
  VF - to end/1 -> Bus Creator/5  "Mode"
  Vcmd pu 1.005 - 1.01/1 -> Bus Creator/3  "V"
  Qfactor/1 -> Bus Creator/2  "Q"
  S Profile/1 -> Pfactor/1, Qfactor/1  "P"
  Bus Creator/1 -> S/1
  DONOTCHANGE/1 -> F/1, V/1, Q/1, P/1

== system MANUAL_INTEGRATION_TEST_01/SC_ctrl/RMS_Calculator1 ==
  s_in : Inport
  Demux : Demux  Outputs=3
  Discrete  Mean value6 : powerlib_extras/Discrete Measurements/Discrete  Mean value  Freq=60  Vinit=0  Ts=Ts
  Mux2 : Mux  Inputs=2
  Product3 : Product  RndMeth=Zero
  Signed Sqrt : Sqrt  SaturateOnIntegerOverflow=on
  s_out : Outport
  wires:
  Demux/1 -> Product3/1, Product3/2
  Product3/1 -> Discrete  Mean value6/1
  Discrete  Mean value6/1 -> Signed Sqrt/1
  s_in/1 -> Mux2/1, Demux/1  "3ph_inst"
  Mux2/1 -> s_out/1  "inst_rms"
  Signed Sqrt/1 -> Mux2/2  "1ph_rms"

== system MANUAL_INTEGRATION_TEST_01/SC_ctrl/RMS_Calculator2 ==
  s_in : Inport
  Demux : Demux  Outputs=3
  Discrete  Mean value6 : powerlib_extras/Discrete Measurements/Discrete  Mean value  Freq=60  Vinit=0  Ts=Ts
  Mux2 : Mux  Inputs=2
  Product3 : Product  RndMeth=Zero
  Signed Sqrt : Sqrt  SaturateOnIntegerOverflow=on
  s_out : Outport
  wires:
  Demux/1 -> Product3/1, Product3/2
  Product3/1 -> Discrete  Mean value6/1
  Discrete  Mean value6/1 -> Signed Sqrt/1
  s_in/1 -> Mux2/1, Demux/1  "3ph_inst"
  Mux2/1 -> s_out/1  "inst_rms"
  Signed Sqrt/1 -> Mux2/2  "1ph_rms"

== system MANUAL_INTEGRATION_TEST_01/SC_ctrl/RMS_Calculator3 ==
  s_in : Inport
  Demux : Demux  Outputs=3
  Discrete  Mean value6 : powerlib_extras/Discrete Measurements/Discrete  Mean value  Freq=60  Vinit=0  Ts=Ts
  Mux2 : Mux  Inputs=2
  Product3 : Product  RndMeth=Zero
  Signed Sqrt : Sqrt  SaturateOnIntegerOverflow=on
  s_out : Outport
  wires:
  Demux/1 -> Product3/1, Product3/2
  Product3/1 -> Discrete  Mean value6/1
  Discrete  Mean value6/1 -> Signed Sqrt/1
  s_in/1 -> Mux2/1, Demux/1  "3ph_inst"
  Mux2/1 -> s_out/1  "inst_rms"
  Signed Sqrt/1 -> Mux2/2  "1ph_rms"

== system MANUAL_INTEGRATION_TEST_01/SC_ctrl/RMS_Calculator4 ==
  s_in : Inport
  Demux : Demux  Outputs=3
  Discrete  Mean value6 : powerlib_extras/Discrete Measurements/Discrete  Mean value  Freq=60  Vinit=0  Ts=Ts
  Mux2 : Mux  Inputs=2
  Product3 : Product  RndMeth=Zero
  Signed Sqrt : Sqrt  SaturateOnIntegerOverflow=on
  s_out : Outport
  wires:
  Demux/1 -> Product3/1, Product3/2
  Product3/1 -> Discrete  Mean value6/1
  Discrete  Mean value6/1 -> Signed Sqrt/1
  s_in/1 -> Mux2/1, Demux/1  "3ph_inst"
  Mux2/1 -> s_out/1  "inst_rms"
  Signed Sqrt/1 -> Mux2/2  "1ph_rms"

== system MANUAL_INTEGRATION_TEST_01/SC_ctrl/RMS_Calculator5 ==
  s_in : Inport
  Demux : Demux  Outputs=3
  Discrete  Mean value6 : powerlib_extras/Discrete Measurements/Discrete  Mean value  Freq=60  Vinit=0  Ts=Ts
  Mux2 : Mux  Inputs=2
  Product3 : Product  RndMeth=Zero
  Signed Sqrt : Sqrt  SaturateOnIntegerOverflow=on
  s_out : Outport
  wires:
  Demux/1 -> Product3/1, Product3/2
  Product3/1 -> Discrete  Mean value6/1
  Discrete  Mean value6/1 -> Signed Sqrt/1
  s_in/1 -> Mux2/1, Demux/1  "3ph_inst"
  Mux2/1 -> s_out/1  "inst_rms"
  Signed Sqrt/1 -> Mux2/2  "1ph_rms"

== system MANUAL_INTEGRATION_TEST_01/SC_ctrl/RMS_Calculator6 ==
  s_in : Inport
  Demux : Demux  Outputs=3
  Discrete  Mean value6 : powerlib_extras/Discrete Measurements/Discrete  Mean value  Freq=60  Vinit=0  Ts=Ts
  Mux2 : Mux  Inputs=2
  Product3 : Product  RndMeth=Zero
  Signed Sqrt : Sqrt  SaturateOnIntegerOverflow=on
  s_out : Outport
  wires:
  Demux/1 -> Product3/1, Product3/2
  Product3/1 -> Discrete  Mean value6/1
  Discrete  Mean value6/1 -> Signed Sqrt/1
  s_in/1 -> Mux2/1, Demux/1  "3ph_inst"
  Mux2/1 -> s_out/1  "inst_rms"
  Signed Sqrt/1 -> Mux2/2  "1ph_rms"

== system MANUAL_INTEGRATION_TEST_01/SC_ctrl/RMS_Calculator7 ==
  s_in : Inport
  Demux : Demux  Outputs=3
  Discrete  Mean value6 : powerlib_extras/Discrete Measurements/Discrete  Mean value  Freq=60  Vinit=0  Ts=Ts
  Mux2 : Mux  Inputs=2
  Product3 : Product  RndMeth=Zero
  Signed Sqrt : Sqrt  SaturateOnIntegerOverflow=on
  s_out : Outport
  wires:
  Demux/1 -> Product3/1, Product3/2
  Product3/1 -> Discrete  Mean value6/1
  Discrete  Mean value6/1 -> Signed Sqrt/1
  s_in/1 -> Mux2/1, Demux/1  "3ph_inst"
  Mux2/1 -> s_out/1  "inst_rms"
  Signed Sqrt/1 -> Mux2/2  "1ph_rms"

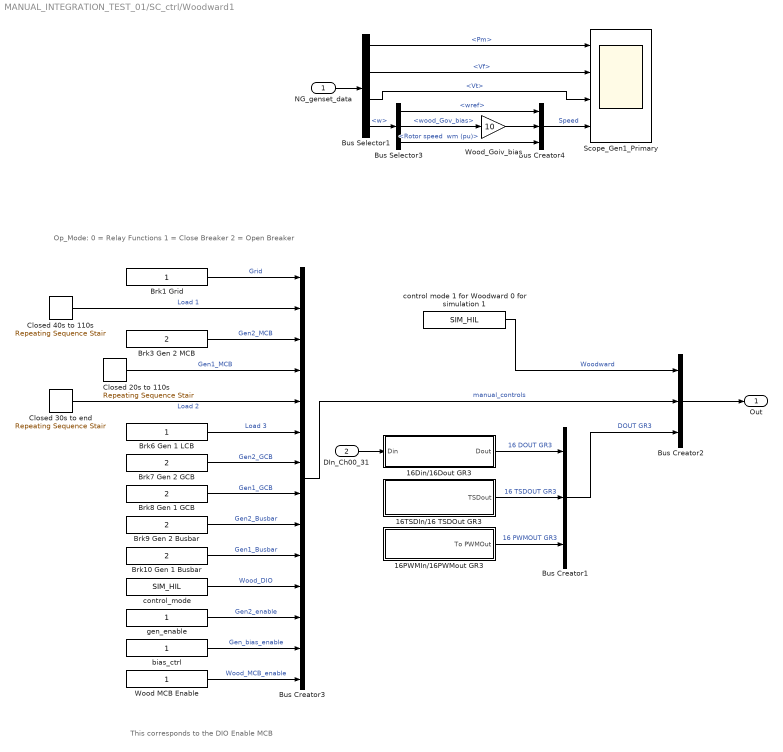
== system MANUAL_INTEGRATION_TEST_01/SC_ctrl/Woodward1 ==
  note: This corresponds to
      | the DIO Enable MCB
  note: Op_Mode:
      | 0 = Relay Functions
      | 1 = Close Breaker
      | 2 = Open Breaker
  NG_genset_data : Inport
  DIn_Ch00_31 : Inport  Port=2
  16Din/16Dout GR3 : Subsystem
  16PWMIn/16PWMout GR3 : Subsystem
  16TSDIn/16 TSDOut GR3 : Subsystem
  Brk1 Grid : Constant
  Brk10 Gen 1 Busbar : Constant  Value=2
  Brk3 Gen 2 MCB : Constant  Value=2
  Brk6 Gen 1 LCB : Constant
  Brk7 Gen 2 GCB : Constant  Value=2
  Brk8 Gen 1 GCB : Constant  Value=2
  Brk9 Gen 2 Busbar : Constant  Value=2
  Bus Creator1 : BusCreator  Inputs=3
  Bus Creator2 : BusCreator  Inputs=3
  Bus Creator3 : BusCreator  Inputs=14
  Bus Creator4 : BusCreator  Inputs=3
  Bus Selector1 : BusSelector  OutputSignals=Pm,Vf,Vt,w
  Bus Selector3 : BusSelector  OutputSignals="wref,w.wood_Gov_bias,w.Rotor speed  wm (pu)"
  Closed 20s to 110s : simulink/Sources/Repeating Sequence Stair  OutValues=[2 2 2 2 1 1 1 1 1 1 1 1 1 1 1 1 1 1 1 1 1 1 2 2 2 2 2]  tsamp=[5 Ts]  OutMin=[]  OutMax=[]  OutDataTypeStr=double  OutputDataTypeScalingMode=double  OutDataType=fixdt(0,8)  ConRadixGroup=Best Precision: Vector-wise  OutScaling=2^-12
  Closed 30s to end : simulink/Sources/Repeating Sequence Stair  OutValues=[2 2 2 2 2 2 1 1 1 1 1 1 1 1 1 1 1 1 1 1 1 1 ]  tsamp=[5 Ts]  OutMin=[]  OutMax=[]  OutDataTypeStr=double  OutputDataTypeScalingMode=double  OutDataType=fixdt(0,8)  ConRadixGroup=Best Precision: Vector-wise  OutScaling=2^-12
  Closed 40s to 110s : simulink/Sources/Repeating Sequence Stair  OutValues=[2 2 2 2 2 2 2 2 1 1 1 1 1 1 1 1 1 1 1 1 1 1 2 2 2]  tsamp=[5 Ts]  OutMin=[]  OutMax=[]  OutDataTypeStr=double  OutputDataTypeScalingMode=double  OutDataType=fixdt(0,8)  ConRadixGroup=Best Precision: Vector-wise  OutScaling=2^-12
  Scope_Gen1_Primary : Scope  NumInputPorts=4
      settings: TimeRange=1  YMin=-0.1~-1~0.9~0.9  YMax=0.7~6~1.2~1.2  SaveName=ScopeData4
  Wood MCB Enable : Constant
  Wood_Goiv_bias : Gain  Gain=10
  bias_ctrl : Constant
  control mode 1 for Woodward 0 for simulation 1 : Constant  Value=SIM_HIL
  control_mode : Constant  Value=SIM_HIL
  gen_enable : Constant
  Out : Outport
  wires:
  Brk1 Grid/1 -> Bus Creator3/1  "Grid"
  Brk10 Gen 1 Busbar/1 -> Bus Creator3/10  "Gen1_Busbar"
  Brk9 Gen 2 Busbar/1 -> Bus Creator3/9  "Gen2_Busbar"
  Wood_Goiv_bias/1 -> Bus Creator4/2
  Brk8 Gen 1 GCB/1 -> Bus Creator3/8  "Gen1_GCB"
  Brk7 Gen 2 GCB/1 -> Bus Creator3/7  "Gen2_GCB"
  Brk6 Gen 1 LCB/1 -> Bus Creator3/6  "Load 3"
  Closed 30s to end/1 -> Bus Creator3/5  "Load 2"
  Bus Creator4/1 -> Scope_Gen1_Primary/4  "Speed"
  Bus Selector3/3 -> Bus Creator4/3  "<Rotor speed  wm (pu)>"
  Bus Selector3/2 -> Wood_Goiv_bias/1  "<wood_Gov_bias>"
  Bus Selector3/1 -> Bus Creator4/1  "<wref>"
  Bus Selector1/4 -> Bus Selector3/1  "<w>"
  Wood MCB Enable/1 -> Bus Creator3/14  "Wood_MCB_enable"
  NG_genset_data/1 -> Bus Selector1/1
  Bus Selector1/3 -> Scope_Gen1_Primary/3  "<Vt>"
  Bus Selector1/2 -> Scope_Gen1_Primary/2  "<Vf>"
  Bus Selector1/1 -> Scope_Gen1_Primary/1  "<Pm>"
  DIn_Ch00_31/1 -> 16Din/16Dout GR3/1(Din)
  Bus Creator2/1 -> Out/1
  bias_ctrl/1 -> Bus Creator3/13  "Gen_bias_enable"
  gen_enable/1 -> Bus Creator3/12  "Gen2_enable"
  control_mode/1 -> Bus Creator3/11  "Wood_DIO"
  Closed 20s to 110s/1 -> Bus Creator3/4  "Gen1_MCB"
  Brk3 Gen 2 MCB/1 -> Bus Creator3/3  "Gen2_MCB"
  Closed 40s to 110s/1 -> Bus Creator3/2  "Load 1"
  Bus Creator3/1 -> Bus Creator2/2  "manual_controls"
  Bus Creator1/1 -> Bus Creator2/3  "DOUT GR3"
  16PWMIn/16PWMout GR3/1(To PWMOut) -> Bus Creator1/3  "16 PWMOUT GR3"
  16TSDIn/16 TSDOut GR3/1(TSDout) -> Bus Creator1/2  "16 TSDOUT GR3"
  16Din/16Dout GR3/1(Dout) -> Bus Creator1/1  "16 DOUT GR3"
  control mode 1 for Woodward 0 for simulation 1/1 -> Bus Creator2/1  "Woodward"

== system MANUAL_INTEGRATION_TEST_01/SM_system/DMSCommandsToMGC ==
  note: All parameters Active "1"
  DSO Command duration : Constant  Value=DSO_Duration
  DSO Command start time : Constant  Value=DSO_Start_Time
  DSO Disconnect/Reconnect Command : Constant  Value=DSO_Disconnect
  DSO Export/Import Command : Constant  Value=DSO_Export
  F3 : Constant  Value=DSO_PF_Support
  "Import/Export Value, kW" : Constant  Value=Import_Export_Value
  "PF Value pu, + (lagging) or - (leading)" : Constant  Value=PF_Value
  VAR Support Command : Constant  Value=DSO_VAR_Support
  "VAR Value, kVAr" : Constant  Value=VAR_Value
  DSO_Start_Time : Outport
  DSO_Duration : Outport  Port=2
  DSO_Disconnect : Outport  Port=3
  DSO_Export : Outport  Port=4
  Import_Export_Value : Outport  Port=5
  DSO_PF_Support : Outport  Port=6
  PF_Value : Outport  Port=7
  DSO_VAR_Support : Outport  Port=8
  VAR_Value : Outport  Port=9
  wires:
  "Import/Export Value, kW"/1 -> Import_Export_Value/1  "Import_Export_Value"
  DSO Command duration/1 -> DSO_Duration/1  "DSO_Duration"
  DSO Command start time/1 -> DSO_Start_Time/1  "DSO_Start_Time"
  "PF Value pu, + (lagging) or - (leading)"/1 -> PF_Value/1  "PF_Value"
  "VAR Value, kVAr"/1 -> VAR_Value/1  "VAR_Value"
  VAR Support Command/1 -> DSO_VAR_Support/1  "DSO_VAR_Support"
  F3/1 -> DSO_PF_Support/1  "DSO_PF_Support"
  DSO Export/Import Command/1 -> DSO_Export/1  "DSO_Export"
  DSO Disconnect/Reconnect Command/1 -> DSO_Disconnect/1  "DSO_Disconnect"

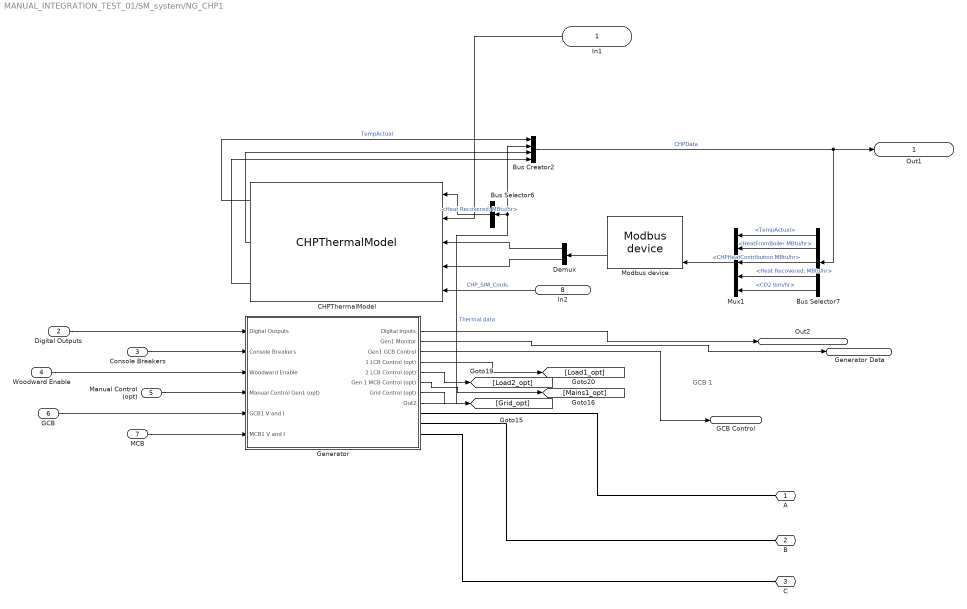
== system MANUAL_INTEGRATION_TEST_01/SM_system/NG_CHP1 ==
  note: GCB 1
  In1 : Inport
  Digital Outputs : Inport  Port=2
  Console Breakers : Inport  Port=3
  Woodward Enable : Inport  Port=4
  Manual Control (opt) : Inport  Port=5
  GCB : Inport  Port=6
  MCB : Inport  Port=7
  In2 : Inport  Port=8
  Bus Creator2 : BusCreator
  Bus Selector6 : BusSelector  OutputSignals=Heat Recovered; MBtu/hr
  Bus Selector7 : BusSelector  OutputSignals=TempActual,HeatFromBoiler MBtu/hr,CHPHeatContribution MBtu/hr,Thermal data.Heat Recovered; MBtu/hr,Thermal data.CO2 lbm/hr
  CHPThermalModel : CHP_Model_lib/CHPThermalModel  SIM_HIL=SIM_HIL
  Demux : Demux  Outputs=2
  Generator : Subsystem  AncestorBlock=NG_Genset_lib/Generator
  Modbus device : rtio_generic_modbus/Modbus device  conf_name=CHP_slave_cfg.opal  conf_name_mask=CHP_slave_cfg.xls  sample_time=Ts
  Mux1 : Mux  Inputs=5
  A : PMIOPort  Tag=A  Port=1  Side=Right
      settings: AttributesFormatString=A
  B : PMIOPort  Port=2  Side=Right
  C : PMIOPort  Port=3  Side=Right
  Out1 : Outport
  Out2 : Outport  Port=2
  Generator Data : Outport  Port=3
  GCB Control : Outport  Port=4
  wires:
  In2/1 -> CHPThermalModel/5  "CHP_SIM_Cmds"
  Generator/1(Digital Inputs) -> Out2/1
  Bus Creator2/1 -> Out1/1, Bus Selector7/1  "CHPData"
  Bus Selector6/1 -> CHPThermalModel/1  "<Heat Recovered; MBtu/hr>"
  Generator/4(1 LCB Control (opt)) -> [Load1_opt]
  Generator/3(Gen1 GCB Control) -> GCB Control/1
  MCB/1 -> Generator/6(MCB1 V and I)
  Generator/5(2 LCB Control (opt)) -> [Load2_opt]
  Manual Control (opt)/1 -> Generator/4(Manual Control Gen1 (opt))
  GCB/1 -> Generator/5(GCB1 V and I)
  Generator/2(Gen1 Monitor) -> Generator Data/1
  Woodward Enable/1 -> Generator/3(Woodward Enable)
  Modbus device/2 -> Demux/1
  Generator/8(Out2) -> Bus Selector6/1, Bus Creator2/2  "Thermal data"
  CHPThermalModel/3 -> Bus Creator2/4
  Demux/1 -> CHPThermalModel/3
  Mux1/1 -> Modbus device/4
  In1/1 -> CHPThermalModel/2
  Bus Selector7/1 -> Mux1/1  "<TempActual>"
  Bus Selector7/4 -> Mux1/4  "<Heat Recovered; MBtu/hr>"
  Bus Selector7/5 -> Mux1/5  "<CO2 lbm/hr>"
  Bus Selector7/2 -> Mux1/2  "<HeatFromBoiler MBtu/hr>"
  Digital Outputs/1 -> Generator/1(Digital Outputs)
  Generator/7(Grid Control (opt)) -> [Grid_opt]
  Console Breakers/1 -> Generator/2(Console Breakers)
  Generator/6(Gen 1 MCB Control (opt)) -> [Mains1_opt]
  CHPThermalModel/2 -> Bus Creator2/3
  Demux/2 -> CHPThermalModel/4
  CHPThermalModel/1 -> Bus Creator2/1  "TempActual"
  Bus Selector7/3 -> Mux1/3  "<CHPHeatContribution MBtu/hr>"
  connections:
  Generator/RConn1 -- A/RConn1
  Generator/RConn2 -- B/RConn1
  Generator/RConn3 -- C/RConn1

== system MANUAL_INTEGRATION_TEST_01/SM_system/TestSequenceCommands ==
  F1 : Constant  Value=fault1
  F10 : Constant  Value=load_gain
  F2 : Constant  Value=fault2
  F3 : Constant  Value=fault3
  F4 : Constant  Value=fault4
  F5 : Constant  Value=fault5
  F6 : Constant  Value=fault6
  F7 : Constant  Value=fault7
  F8 : Constant  Value=fault8
  Fault1 : Outport
  Fault2 : Outport  Port=2
  Fault3 : Outport  Port=3
  Fault4 : Outport  Port=4
  Fault5 : Outport  Port=5
  Fault6 : Outport  Port=6
  Fault7 : Outport  Port=7
  "Fault8 " : Outport  Port=8
  loads : Outport  Port=9
  wires:
  F10/1 -> loads/1
  F7/1 -> Fault7/1
  F6/1 -> Fault6/1
  F8/1 -> "Fault8 "/1
  F5/1 -> Fault5/1
  F4/1 -> Fault4/1
  F3/1 -> Fault3/1
  F2/1 -> Fault2/1
  F1/1 -> Fault1/1
